simulink model "Y6MultirotorMPCSimulation"  (R2019b)
settings: Solver=FixedStepAuto  StartTime=0.0  StopTime=60  RelTol=1e-3
values from neighbouring files (symbols this model uses):
  Time = 100    [Simulation.m]
undefined symbols (not defined in the file or in its folder): Cr, DiscIntNeverNeededParam, Discrete, Kdt, Kidt, N, Rv, T, U_e
libraries: ctrlSharedLib x1, mpclib x1
settings Model: Creator=oscar  LastModifiedBy=alexd
settings SolverCC: AlgebraicLoopSolver=LineSearch
settings DataIOCC: ReturnWorkspaceOutputs=off
settings OptimizationCC: OptimizeBlockIOStorage=off  BufferReuse=off  GlobalBufferReuse=off  ExpressionFolding=off  LocalBlockOutputs=off  OptimizeDataStoreBuffers=off  BusAssignmentInplaceUpdate=off
settings DebuggingCC: SFUnexpectedBacktrackingDiag=warning  SFNoUnconditionalDefaultTransitionDiag=warning  ArithmeticOperatorsInVariantConditions=warning
settings SFSimCC: SimUseLocalCustomCode=off  CustomCodeUndefinedFunction=UseInterfaceOnly
settings RTWCC: GenCodeOnly=on  GenerateReport=on  RTWUseLocalCustomCode=off  BuildConfiguration=Debug  LaunchReport=on
settings CodeAppCC: ForceParamTrailComments=on  MATLABSourceComments=on  EnableCustomComments=on
settings GRTTargetCC: CombineSignalStateStructs=on  SupportVariableSizeSignals=on  MultiInstanceErrorCode=Warning

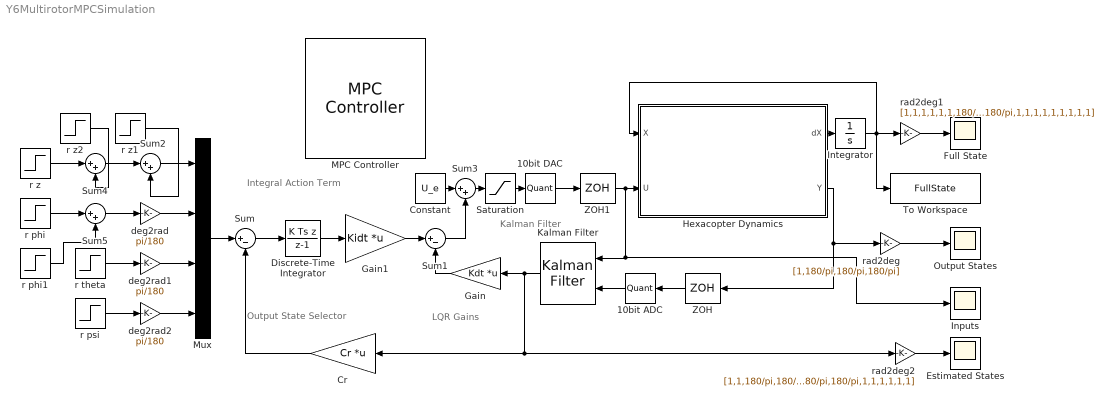
== system Y6MultirotorMPCSimulation ==
  note: LQR Gains
  note: Kalman Filter
  note: Integral Action Term
  note: Output State Selector
  10bit ADC : Quantizer  QuantizationInterval=3.3/((2^10)-1)
  10bit DAC : Quantizer  QuantizationInterval=3.3/((2^10)-1)
  Constant : Constant  Value=U_e
  Cr : Gain  Gain=Cr  Multiplication=Matrix(K*u)
  Discrete-Time Integrator : DiscreteIntegrator  IntegratorMethod=Integration: Backward Euler  gainval=1/T  SampleTime=T  ICPrevOutput=DiscIntNeverNeededParam  ICPrevScaledInput=DiscIntNeverNeededParam
  Estimated States : Scope
  Full State : Scope
  Gain : Gain  Gain=Kdt  Multiplication=Matrix(K*u)
  Gain1 : Gain  Gain=Kidt  Multiplication=Matrix(K*u)
  Hexacopter Dynamics : MATLAB Function  TreatAsAtomicUnit=on
  Inputs : Scope
  Integrator : Integrator  InitialCondition=[0;0;0;0;0;0;0;0;0;0;0;0;0;0;0;0;0;0]
  Kalman Filter : ctrlSharedLib/Kalman Filter  TimeDomain=Discrete-Time  UseCurrentEstimator=on  ModelSource=LTI State-Space Variable  ModelSourceVariable=sysdt  A=0.95  B=1  C=1  D=0  NumberOfStates=1  NumberOfInputs=1  NumberOfOutputs=1  InitialEstimateSource=Dialog  X0=0  P0=10  UseK=off  UseGH=off  NumberOfProcessNoiseInputs=1  G=1  TimeInvariantG=on  H=0  TimeInvariantH=on  Q=Rw  TimeInvariantQ=on  R=Rv  TimeInvariantR=on  N=N  TimeInvariantN=on  AddInputPort=on  AddEnablePort=off  OutputEstimatedY=off  OutputP=off  Ts=-1
      settings: SourceProductBaseCode=CT
  MPC Controller : mpclib/MPC Controller  SCDEnableBlockLinearizationSpecification=on  is_multiple=0  enable_value=0  return_u0=off  updateMPCinCallerWorkspace=on  md_inport=on  mv_inport=off  uref_inport=off  return_cost=off  return_mvseq=off  return_qpstatus=off  return_xseq=off  return_state=off  return_ovseq=off  state_inport=off  umin_inport=off  umax_inport=off  ymin_inport=off  ymax_inport=off  cc_inport=off  ywt_inport=off  uwt_inport=off  duwt_inport=off  rhoeps_inport=off  pm_inport=off  MaximumP=10  HorizonChoice=FixedHorizon  n_ts=1  n_p=10  n_mv=1  n_md=1  n_ud=0  n_mo=1  n_uo=0  BlockDataType=double  SampleTimeInherited=off  switch_inport=off
  Mux : Mux
  Output States : Scope
  Saturation : Saturate  UpperLimit=800  LowerLimit=0
  Sum : Sum  Inputs=|+-
  Sum1 : Sum  Inputs=|+-
  Sum{2..5} (4 alike) : Sum  Inputs=|++
  To Workspace : ToWorkspace  VariableName=FullState  SaveFormat=Timeseries  SampleTime=-1
  ZOH : ZeroOrderHold  SampleTime=T
  ZOH1 : ZeroOrderHold  SampleTime=T
  deg2rad : Gain  Gain=pi/180  SaturateOnIntegerOverflow=on  OutDataTypeStr=Inherit: Same as input  ParamDataTypeStr=Inherit: Same as input
  deg2rad1 : Gain  Gain=pi/180  SaturateOnIntegerOverflow=on  OutDataTypeStr=Inherit: Same as input  ParamDataTypeStr=Inherit: Same as input
  deg2rad2 : Gain  Gain=pi/180  SaturateOnIntegerOverflow=on  OutDataTypeStr=Inherit: Same as input  ParamDataTypeStr=Inherit: Same as input
  r phi : Step  Time=40  After=5  SampleTime=0
  r phi1 : Step  Time=42  After=-5  SampleTime=0
  r psi : Step  Time=0  After=0  SampleTime=0
  r theta : Step  Time=0  After=0  SampleTime=0
  r z : Step  Time=10  SampleTime=0
  r z1 : Step  Time=30  After=-1  SampleTime=0
  r z2 : Step  Time=20  SampleTime=0
  rad2deg : Gain  Gain=[1,180/pi,180/pi,180/pi]  SaturateOnIntegerOverflow=on  OutDataTypeStr=Inherit: Same as input  ParamDataTypeStr=Inherit: Same as input
  rad2deg1 : Gain  Gain=[1,1,1,1,1,1,180/pi,180/pi,180/pi,1,1,1,1,1,1,1,1,1]  SaturateOnIntegerOverflow=on  OutDataTypeStr=Inherit: Same as input  ParamDataTypeStr=Inherit: Same as input
  rad2deg2 : Gain  Gain=[1,1,180/pi,180/pi,180/pi,180/pi,180/pi,180/pi,1,1,1,1,1,1]  SaturateOnIntegerOverflow=on  OutDataTypeStr=Inherit: Same as input  ParamDataTypeStr=Inherit: Same as input
  wires:
  Hexacopter Dynamics/1(dX) -> Integrator/1
  Integrator/1 -> rad2deg1/1, Hexacopter Dynamics/1(X), To Workspace/1
  Kalman Filter/1 -> rad2deg2/1, Cr/1, Gain/1
  Gain/1 -> Sum1/2
  Gain1/1 -> Sum1/1
  Hexacopter Dynamics/2(Y) -> rad2deg/1, ZOH/1
  Constant/1 -> Sum3/1
  deg2rad/1 -> Mux/2
  r theta/1 -> deg2rad1/1
  r psi/1 -> deg2rad2/1
  deg2rad2/1 -> Mux/4
  deg2rad1/1 -> Mux/3
  rad2deg/1 -> Output States/1
  rad2deg1/1 -> Full State/1
  Sum3/1 -> Saturation/1
  Sum/1 -> Discrete-Time Integrator/1
  Discrete-Time Integrator/1 -> Gain1/1
  Cr/1 -> Sum/2
  Sum1/1 -> Sum3/2
  Saturation/1 -> 10bit DAC/1
  ZOH/1 -> 10bit ADC/1
  Mux/1 -> Sum/1
  10bit ADC/1 -> Kalman Filter/2
  Sum2/1 -> Mux/1
  r z1/1 -> Sum2/2
  r z/1 -> Sum4/1
  r z2/1 -> Sum4/2
  Sum4/1 -> Sum2/1
  Sum5/1 -> deg2rad/1
  r phi/1 -> Sum5/1
  r phi1/1 -> Sum5/2
  rad2deg2/1 -> Estimated States/1
  10bit DAC/1 -> ZOH1/1
  ZOH1/1 -> Inputs/1, Kalman Filter/1, Hexacopter Dynamics/2(U)

== matlab function Y6MultirotorMPCSimulation/Hexacopter Dynamics ==
  data: dX output; X input; U input; Y output
function [dX,Y]  = Hexacopter_Dynamics(X,U)
%% Mass of the Multirotor in Kilograms as taken from the CAD

M = 1.455882; 
g = 9.81;

%% Dimensions of Multirotor

L1 = 19/100; % along X-axis Distance from left and right motor pair to center of mass
L2 = 18/100; % along Y-axis Vertical Distance from left and right motor pair to center of mass
L3 = 30/100; % along Y-axis Distance from motor pair to center of mass

%%  Mass Moment of Inertia as Taken from the CAD
% Inertia Matrix and Diagolalisation CAD model coordinate system rotated 90 degrees about X

Ixx = 0.014;
Iyy = 0.028;
Izz = 0.038;

%% Motor Thrust and Torque Constants (To be determined experimentally)

Kw = 0.85;
Ktau =  7.708e-10;
Kthrust =  1.812e-07;
Kthrust2 = 0.0007326;
Mtau = (1/44.22);
Ku = 515.5*Mtau;

%% Air resistance damping coeeficients

Dxx = 0.01212;
Dyy = 0.01212;
Dzz = 0.0648;                          

%% X = [x xdot y ydot z zdot phi phidot theta thetadot psi psidot w1 w2 w3 w4 w5 w6]

x = X(1);
xdot = X(2);
y = X(3);
ydot = X(4);
z = X(5);
zdot = X(6);

phi = X(7); 
theta = X(8);
psi = X(9);

p = X(10);
q = X(11);
r = X(12);

w1 = X(13);
w2 = X(14);
w3 = X(15);
w4 = X(16);
w5 = X(17);
w6 = X(18);

%% Initialise Outputs

dX = zeros(18,1);
Y = zeros(4,1);

%% Motor Dynamics: dX = [w1dot w2dot w3dot w4dot w5dot w6dot], U = Duty Cycle of the pwm signal 0-100%

dX(13) = -(1/Mtau)*w1 + Ku/Mtau*U(1);
dX(14) = -(1/Mtau)*w2 + Ku/Mtau*U(2);
dX(15) = -(1/Mtau)*w3 + Ku/Mtau*U(3);
dX(16) = -(1/Mtau)*w4 + Ku/Mtau*U(4);
dX(17) = -(1/Mtau)*w5 + Ku/Mtau*U(5);
dX(18) = -(1/Mtau)*w6 + Ku/Mtau*U(6);

%% Motor Forces and Torques

F = zeros(6,1);
T = zeros(6,1);

F(1)= Kw*Kthrust*(w1^2) + Kthrust2*w1;
F(2)= Kthrust*(w2^2) + Kthrust2*w2;
F(3)= Kw*Kthrust*(w3^2)+ Kthrust2*w3;
F(4)= Kthrust*(w4^2) + Kthrust2*w4;
F(5)= Kw*Kthrust*(w5^2) + Kthrust2*w5;
F(6)= Kthrust*(w6^2) + Kthrust2*w6;

T(1)= -Ktau*(w1^2);
T(2)= Ktau*(w2^2);
T(3)= Ktau*(w3^2);
T(4)= -Ktau*(w4^2);
T(5)= -Ktau*(w5^2);
T(6)= Ktau*(w6^2);

Fn = sum(F);
Tn = sum(T);

%% First Order Direvatives dX = [xdot ydot zdot phidot thetadot psidot]

dX(1) = X(2);
dX(3) = X(4);
dX(5) = X(6);
dX(7) = p + q*(sin(phi)*tan(theta)) + r*(cos(phi)*tan(theta));
dX(8) = q*cos(phi) - r*sin(phi);
dX(9) = q*(sin(phi)/cos(theta)) + r*(cos(phi)/cos(theta));

%% Second Order Direvatives: dX = [xddot yddot zddot pdot qdot rdot]

dX(2) = Fn/M*(cos(phi)*sin(theta)*cos(psi)) + Fn/M*(sin(phi)*sin(psi)) - (Dxx/M)*xdot;
dX(4) = Fn/M*(cos(phi)*sin(theta)*sin(psi)) - Fn/M*(sin(phi)*cos(psi)) - (Dyy/M)*ydot;
dX(6) = Fn/M*(cos(phi)*cos(theta)) - g - (Dzz/M)*zdot;

dX(10) = (L1/Ixx)*((F(1)+F(2)) - (F(3)+F(4))) - ((Izz-Iyy)/Ixx)*(r*q); 
dX(11) = (L3/Iyy)*(F(5)+F(6)) - (L2/Iyy)*(F(1)+F(2)+F(3)+F(4)) - ((Izz-Ixx)/Iyy)*(p*r);
dX(12) = Tn/Izz - ((Iyy-Ixx)/Izz)*(p*q);

%% Measured States

Y(1) = z;
Y(2) = phi;
Y(3) = theta;
Y(4) = psi;

end
